simulink model "crazyflie_simulation"  (R2019a)
settings: Solver=FixedStepAuto  StartTime=0.0  StopTime=100  FixedStep=Ts  RelTol=1e-3
undefined symbols (not defined in the file): b, D_0, D_1, D_2, DiscIntNeverNeededParam, g, I_CF_1, I_CF_1_inv, I_rzz, k_f, k_m, kx, ky, kz, l, m_CF, N_0, N_1, N_2, omegaR_init, T, T_init, Ts
libraries: sharedutil x2, simulink x1
settings Model: Creator=evgheniivolodscoi  LastModifiedBy=evgheniivolodscoi

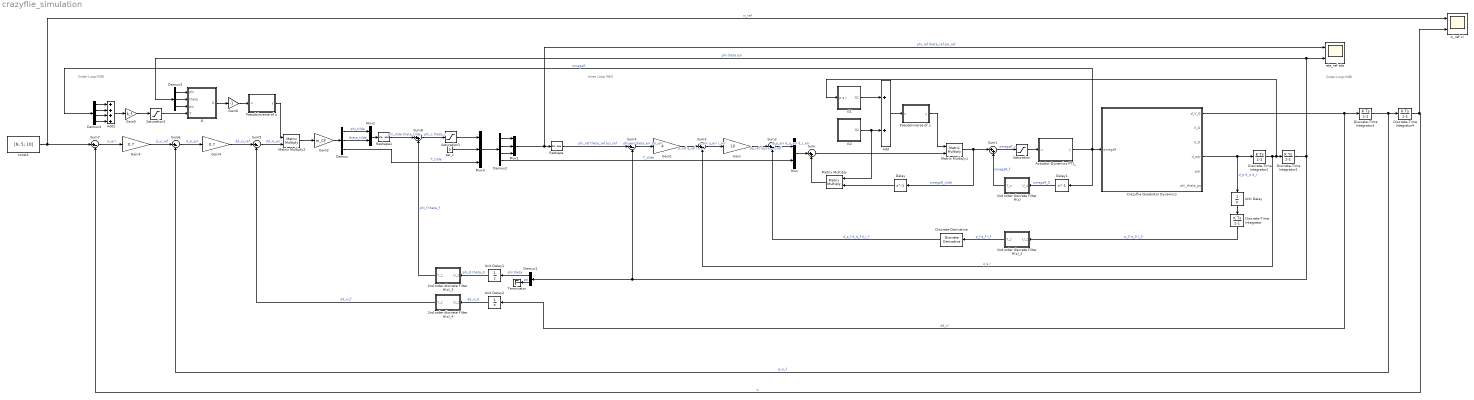
== system crazyflie_simulation ==
  note: Outer Loop INDI
  note: Outer Loop INDI
  note: Inner Loop INDI
  2nd order discrete Filter H(z) : Subsystem
  2nd order discrete Filter H(z)_2 : Subsystem
  2nd order discrete Filter H(z)_3 : Subsystem
  2nd order discrete Filter H(z)_4 : Subsystem
  "Actuator Dynamics PT1_ " : Subsystem
  Add : Sum
  Add1 : Sum  Inputs=++++
  Crazyflie Quadrotor Dynamics : Subsystem
  Delay : Delay  DelayLength=1  InitialCondition=0
  Delay1 : Delay  DelayLength=1  InitialCondition=0
  Demux : Demux  Outputs=3
  Demux1 : Demux  Outputs=2
  Demux2 : Demux
  Demux3 : Demux  Outputs=3
  Demux4 : Demux
  Discrete Derivative : simulink/Discrete/Discrete Derivative  gainval=1.0  ICPrevScaledInput=0.0  OutMin=[]  OutMax=[]  OutDataType=fixdt(1, 16)  OutScaling=2^-10  DoSatur=off
  Discrete-Time Integrator{,1..4} (5 alike) : DiscreteIntegrator  SampleTime=-1  ICPrevOutput=DiscIntNeverNeededParam  ICPrevScaledInput=DiscIntNeverNeededParam
  G : Subsystem
  G1 : Subsystem
  G2 : Subsystem
  Gain : Gain  Gain=10
  Gain1 : Gain  Gain=4
  Gain2 : Gain  Gain=m_CF
  Gain3 : Gain  Gain=0.7
  Gain4 : Gain  Gain=0.7
  Gain5 : Gain  Gain=k_f
  Gain6 : Gain  Gain=-1
  Matrix Multiply : Product  Multiplication=Matrix(*)
  Matrix Multiply1 : Product  Multiplication=Matrix(*)
  Matrix Multiply2 : Product  Multiplication=Matrix(*)
  Mux : Mux  Inputs=2
  Mux1 : Mux  Inputs=3
  Mux2 : Mux  Inputs=2
  Mux3 : Mux  Inputs=3
  Pseudoinverse of u : MATLAB Function  TreatAsAtomicUnit=on
  "Pseudoinverse of u " : MATLAB Function  TreatAsAtomicUnit=on
  Reshape : Reshape  OutputDimensionality=Column vector (2-D)
  Reshape1 : Reshape  OutputDimensionality=Column vector (2-D)
  Saturation : Saturate  UpperLimit=1000  LowerLimit=0
  Saturation1 : Saturate  UpperLimit=60/180*pi  LowerLimit=-60/180*pi
  Saturation2 : Saturate  UpperLimit=inf  LowerLimit=T_init
  Sum : Sum  Inputs=|++
  Sum1 : Sum  Inputs=|++
  Sum{2..7} (6 alike) : Sum  Inputs=|+-
  Sum8 : Sum  Inputs=|++
  Terminator : Terminator
  Unit Delay : UnitDelay  SampleTime=-1  HasFrameUpgradeWarning=on
  Unit Delay1 : UnitDelay  SampleTime=-1  HasFrameUpgradeWarning=on
  Unit Delay2 : UnitDelay  SampleTime=-1  HasFrameUpgradeWarning=on
  const1 : Constant  Value=[6; 5; 10]
  eta_ref eta : Scope  NumInputPorts=2
  psi_c : Constant  Value=0
  xi_ref xi : Scope  NumInputPorts=2
  wires:
  G1/1(G1) -> Add/1
  G2/1(G2) -> Matrix Multiply/1, Add/2
  Matrix Multiply1/1 -> Sum1/1, Delay/1  "omegaR_tilde"
  Delay/1 -> Matrix Multiply/2
  Matrix Multiply/1 -> Sum/2
  Sum/1 -> Matrix Multiply1/2
  Mux/1 -> Sum/1
  Sum1/1 -> Saturation/1  "omegaR_c"
  2nd order discrete Filter H(z)/1(Y_z) -> Sum1/2  "omegaR_f"
  Delay1/1 -> 2nd order discrete Filter H(z)/1(U_z)  "omegaR_0"
  "Actuator Dynamics PT1_ "/1(y) -> Demux4/1, Delay1/1, Crazyflie Quadrotor Dynamics/1(omegaR)  "omegaR"
  Add/1 -> Pseudoinverse of u/1(u)
  Sum2/1 -> Mux/1  "d_p_err d_q_err d_r_err"
  Discrete Derivative/1 -> Sum2/2  "d_p_f d_q_f d_r_f"
  Gain/1 -> Sum2/1  "dp_ref dq_ref dr_ref"
  Sum3/1 -> Gain/1  "p_err q_err r_err"
  Gain1/1 -> Sum3/1  "p_ref q_ref r_ref"
  Discrete-Time Integrator1/1 -> Sum3/2, G1/1(p q r), Discrete-Time Integrator2/1  "p q r"
  Sum4/1 -> Gain1/1  "phi_err theta_err psi_err"
  Discrete-Time Integrator/1 -> 2nd order discrete Filter H(z)_2/1(U_z)  "p_0 q_0 r_0"
  2nd order discrete Filter H(z)_2/1(Y_z) -> Discrete Derivative/1  "p_f q_f r_f"
  Crazyflie Quadrotor Dynamics/4(d_pqr) -> Discrete-Time Integrator1/1, Unit Delay/1  "d_p d_q d_r"
  Unit Delay/1 -> Discrete-Time Integrator/1
  Gain2/1 -> Demux/1
  Sum5/1 -> Matrix Multiply2/2  "dd_xi_err"
  Gain4/1 -> Sum5/1  "dd_xi_ref"
  Gain3/1 -> Sum6/1  "d_xi_ref"
  Sum7/1 -> Gain3/1  "xi_err"
  Discrete-Time Integrator4/1 -> xi_ref xi/2, Sum7/2  "xi"
  const1/1 -> Sum7/1, xi_ref xi/1  "xi_ref"
  Matrix Multiply2/1 -> Gain2/1
  Reshape1/1 -> Sum8/1  "phi_tilde theta_tilde"
  2nd order discrete Filter H(z)_3/1(Y_z) -> Sum8/2  "phi_f theta_f"
  Sum8/1 -> Saturation1/1  "phi_c theta_c"
  Unit Delay1/1 -> 2nd order discrete Filter H(z)_3/1(U_z)  "phi_0 theta_0"
  Demux1/1 -> Unit Delay1/1  "phi theta"
  Demux1/2 -> Terminator/1  "psi"
  Crazyflie Quadrotor Dynamics/1(d_V_O) -> Unit Delay2/1, Discrete-Time Integrator3/1  "dd_xi"
  Discrete-Time Integrator2/1 -> eta_ref eta/2, Demux3/1, Demux1/1, Sum4/2  "phi theta psi"
  Mux1/1 -> eta_ref eta/1, Reshape/1  "phi_ref theta_ref psi_ref"
  Demux2/2 -> Mux1/2
  Demux2/1 -> Mux1/1
  Demux2/3 -> Mux1/3
  Demux2/4 -> Mux/2  "T_tilde"
  Reshape/1 -> Sum4/1  "phi_ref theta_ref psi_ref"
  Pseudoinverse of u/1(y) -> Matrix Multiply1/1
  Demux/1 -> Mux2/1  "phi_tilde"
  Demux/2 -> Mux2/2  "theta_tilde"
  Demux/3 -> Mux3/3  "T_tilde"
  Mux2/1 -> Reshape1/1
  psi_c/1 -> Mux3/2
  Mux3/1 -> Demux2/1
  "Pseudoinverse of u "/1(y) -> Matrix Multiply2/1
  Demux3/1 -> G/1(phi)
  Demux3/2 -> G/2(theta)
  Demux3/3 -> G/3(psi)
  Demux4/1 -> Add1/1
  Demux4/2 -> Add1/2
  Demux4/3 -> Add1/3
  Demux4/4 -> Add1/4
  Add1/1 -> Gain5/1
  Gain5/1 -> Saturation2/1
  2nd order discrete Filter H(z)_4/1(Y_z) -> Sum5/2  "dd_xi_f"
  Unit Delay2/1 -> 2nd order discrete Filter H(z)_4/1(U_z)  "dd_xi_0"
  Discrete-Time Integrator3/1 -> Sum6/2, Discrete-Time Integrator4/1  "d_xi_f"
  Sum6/1 -> Gain4/1  "d_xi_err"
  G/1(G) -> Gain6/1
  Saturation/1 -> "Actuator Dynamics PT1_ "/1(u)
  Saturation1/1 -> Mux3/1
  Saturation2/1 -> G/4(T)
  Gain6/1 -> "Pseudoinverse of u "/1(u)

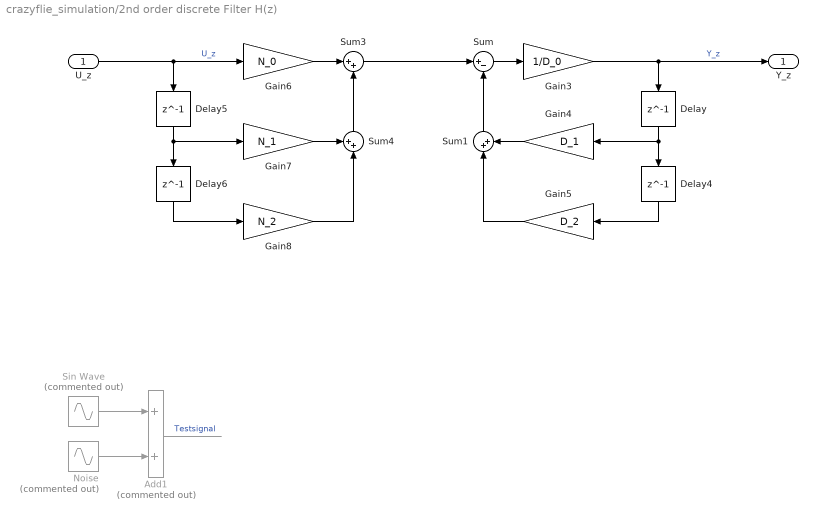
== system crazyflie_simulation/2nd order discrete Filter H(z) ==
  U_z : Inport
  Add1 : Sum  Commented=on
  Delay{,4..6} (4 alike) : Delay  DelayLength=1  InitialCondition=0
  Gain3 : Gain  Gain=1/D_0
  Gain4 : Gain  Gain=D_1
  Gain5 : Gain  Gain=D_2
  Gain6 : Gain  Gain=N_0
  Gain7 : Gain  Gain=N_1
  Gain8 : Gain  Gain=N_2
  Noise : Sin  Commented=on  Amplitude=0.15  Frequency=10*2*pi  SampleTime=0
  Sin Wave : Sin  Commented=on  Frequency=100/2/pi*2*pi  SampleTime=0
  Sum : Sum  Inputs=|+-
  Sum1 : Sum  Inputs=|++
  Sum3 : Sum  Inputs=|++
  Sum4 : Sum  Inputs=++|
  Y_z : Outport
  wires:
  Add1/1 -> ?  "Testsignal"
  Sin Wave/1 -> Add1/1
  Noise/1 -> Add1/2
  Delay6/1 -> Gain8/1
  Gain8/1 -> Sum4/2
  Sum4/1 -> Sum3/2
  Gain7/1 -> Sum4/1
  Delay5/1 -> Gain7/1, Delay6/1
  U_z/1 -> Gain6/1, Delay5/1  "U_z"
  Gain6/1 -> Sum3/1
  Sum3/1 -> Sum/1
  Gain5/1 -> Sum1/1
  Gain4/1 -> Sum1/2
  Gain3/1 -> Delay/1, Y_z/1  "Y_z"
  Sum1/1 -> Sum/2
  Delay4/1 -> Gain5/1
  Delay/1 -> Gain4/1, Delay4/1
  Sum/1 -> Gain3/1

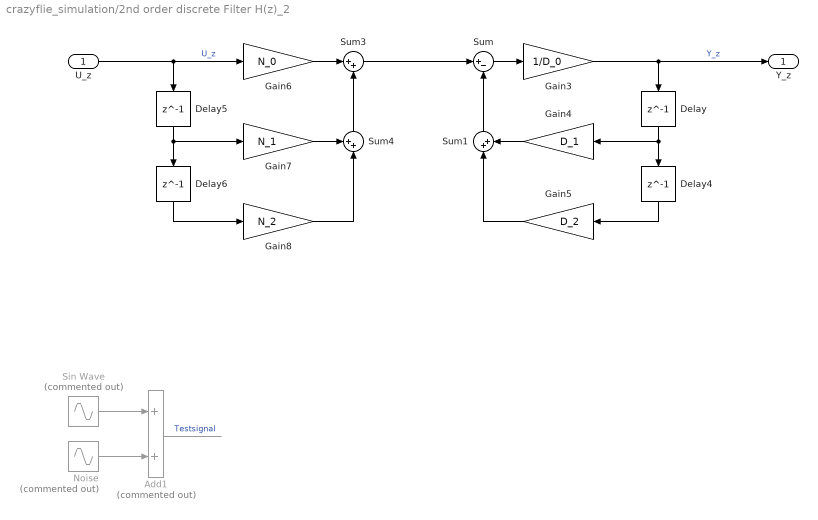
== system crazyflie_simulation/2nd order discrete Filter H(z)_2 ==
  U_z : Inport
  Add1 : Sum  Commented=on
  Delay{,4..6} (4 alike) : Delay  DelayLength=1  InitialCondition=0
  Gain3 : Gain  Gain=1/D_0
  Gain4 : Gain  Gain=D_1
  Gain5 : Gain  Gain=D_2
  Gain6 : Gain  Gain=N_0
  Gain7 : Gain  Gain=N_1
  Gain8 : Gain  Gain=N_2
  Noise : Sin  Commented=on  Amplitude=0.15  Frequency=10*2*pi  SampleTime=0
  Sin Wave : Sin  Commented=on  Frequency=100/2/pi*2*pi  SampleTime=0
  Sum : Sum  Inputs=|+-
  Sum1 : Sum  Inputs=|++
  Sum3 : Sum  Inputs=|++
  Sum4 : Sum  Inputs=++|
  Y_z : Outport
  wires:
  Sum/1 -> Gain3/1
  Delay/1 -> Delay4/1, Gain4/1
  Delay4/1 -> Gain5/1
  Sum1/1 -> Sum/2
  Gain3/1 -> Y_z/1, Delay/1  "Y_z"
  Gain4/1 -> Sum1/2
  Gain5/1 -> Sum1/1
  Sum3/1 -> Sum/1
  Gain6/1 -> Sum3/1
  U_z/1 -> Delay5/1, Gain6/1  "U_z"
  Delay5/1 -> Delay6/1, Gain7/1
  Gain7/1 -> Sum4/1
  Sum4/1 -> Sum3/2
  Gain8/1 -> Sum4/2
  Delay6/1 -> Gain8/1
  Noise/1 -> Add1/2
  Sin Wave/1 -> Add1/1
  Add1/1 -> ?  "Testsignal"

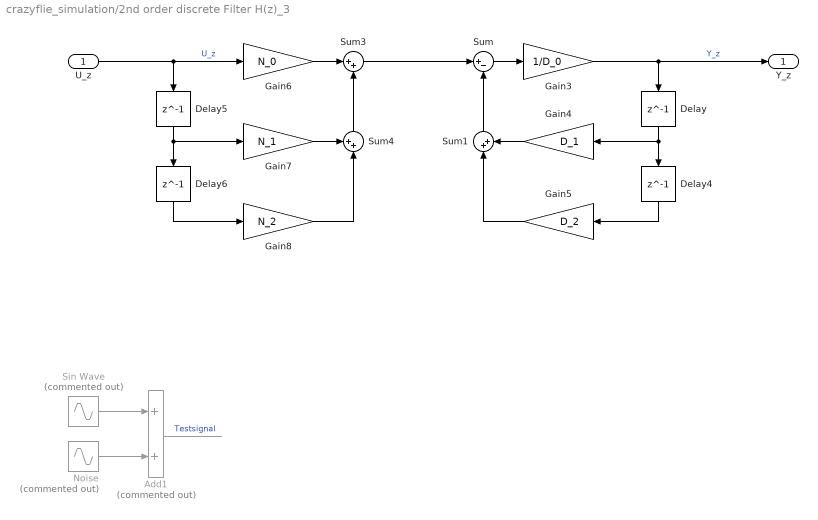
== system crazyflie_simulation/2nd order discrete Filter H(z)_3 ==
  U_z : Inport
  Add1 : Sum  Commented=on
  Delay{,4..6} (4 alike) : Delay  DelayLength=1  InitialCondition=0
  Gain3 : Gain  Gain=1/D_0
  Gain4 : Gain  Gain=D_1
  Gain5 : Gain  Gain=D_2
  Gain6 : Gain  Gain=N_0
  Gain7 : Gain  Gain=N_1
  Gain8 : Gain  Gain=N_2
  Noise : Sin  Commented=on  Amplitude=0.15  Frequency=10*2*pi  SampleTime=0
  Sin Wave : Sin  Commented=on  Frequency=100/2/pi*2*pi  SampleTime=0
  Sum : Sum  Inputs=|+-
  Sum1 : Sum  Inputs=|++
  Sum3 : Sum  Inputs=|++
  Sum4 : Sum  Inputs=++|
  Y_z : Outport
  wires:
  Add1/1 -> ?  "Testsignal"
  Sin Wave/1 -> Add1/1
  Noise/1 -> Add1/2
  Delay6/1 -> Gain8/1
  Gain8/1 -> Sum4/2
  Sum4/1 -> Sum3/2
  Gain7/1 -> Sum4/1
  Delay5/1 -> Gain7/1, Delay6/1
  U_z/1 -> Gain6/1, Delay5/1  "U_z"
  Gain6/1 -> Sum3/1
  Sum3/1 -> Sum/1
  Gain5/1 -> Sum1/1
  Gain4/1 -> Sum1/2
  Gain3/1 -> Delay/1, Y_z/1  "Y_z"
  Sum1/1 -> Sum/2
  Delay4/1 -> Gain5/1
  Delay/1 -> Gain4/1, Delay4/1
  Sum/1 -> Gain3/1

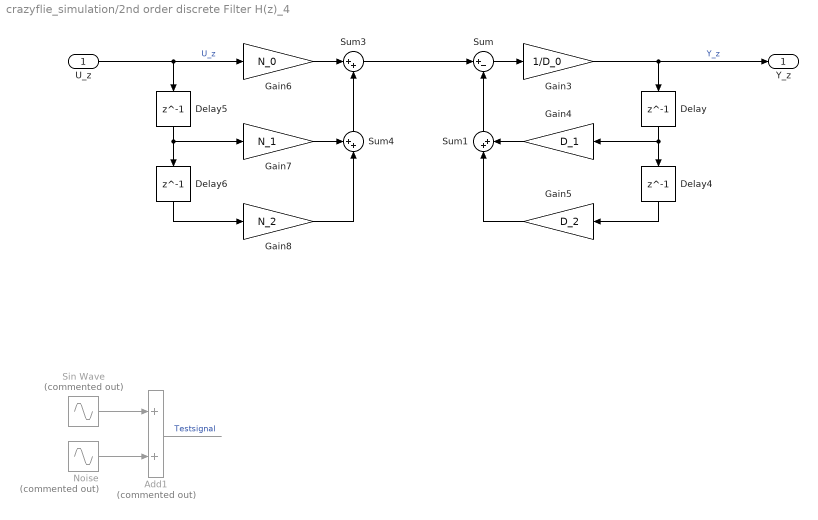
== system crazyflie_simulation/2nd order discrete Filter H(z)_4 ==
  U_z : Inport
  Add1 : Sum  Commented=on
  Delay{,4..6} (4 alike) : Delay  DelayLength=1  InitialCondition=0
  Gain3 : Gain  Gain=1/D_0
  Gain4 : Gain  Gain=D_1
  Gain5 : Gain  Gain=D_2
  Gain6 : Gain  Gain=N_0
  Gain7 : Gain  Gain=N_1
  Gain8 : Gain  Gain=N_2
  Noise : Sin  Commented=on  Amplitude=0.15  Frequency=10*2*pi  SampleTime=0
  Sin Wave : Sin  Commented=on  Frequency=100/2/pi*2*pi  SampleTime=0
  Sum : Sum  Inputs=|+-
  Sum1 : Sum  Inputs=|++
  Sum3 : Sum  Inputs=|++
  Sum4 : Sum  Inputs=++|
  Y_z : Outport
  wires:
  Sum/1 -> Gain3/1
  Delay/1 -> Delay4/1, Gain4/1
  Delay4/1 -> Gain5/1
  Sum1/1 -> Sum/2
  Gain3/1 -> Y_z/1, Delay/1  "Y_z"
  Gain4/1 -> Sum1/2
  Gain5/1 -> Sum1/1
  Sum3/1 -> Sum/1
  Gain6/1 -> Sum3/1
  U_z/1 -> Delay5/1, Gain6/1  "U_z"
  Delay5/1 -> Delay6/1, Gain7/1
  Gain7/1 -> Sum4/1
  Sum4/1 -> Sum3/2
  Gain8/1 -> Sum4/2
  Delay6/1 -> Gain8/1
  Noise/1 -> Add1/2
  Sin Wave/1 -> Add1/1
  Add1/1 -> ?  "Testsignal"

== system crazyflie_simulation/Actuator Dynamics PT1_  ==
  u : Inport
  Gain : Gain  Gain=1/T
  Integrator : Integrator  InitialCondition=omegaR_init
  Sum : Sum  Inputs=|+-
  y : Outport
  wires:
  Sum/1 -> Gain/1
  Gain/1 -> Integrator/1  "d_y"
  u/1 -> Sum/1
  Integrator/1 -> y/1, Sum/2  "y"

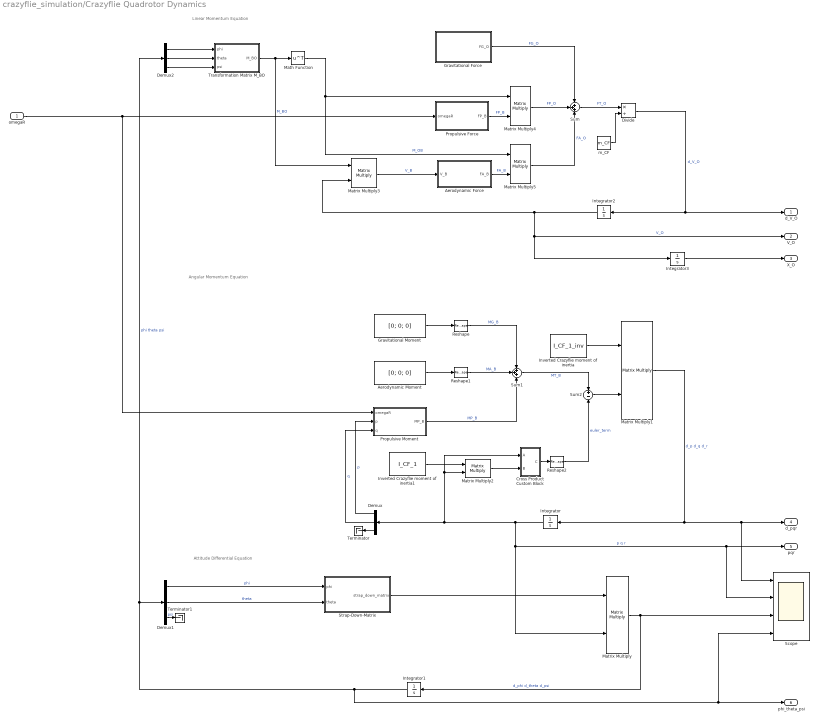
== system crazyflie_simulation/Crazyflie Quadrotor Dynamics ==
  note: Attitude Differential Equation
  note: Angular Momentum Equation
  note: Linear Momentum Equation
  omegaR : Inport
  Aerodynamic Force : Subsystem
  Aerodynamic Moment : Constant  Value=[0; 0; 0]
  Cross Product Custom Block : Subsystem
  Demux : Demux  Outputs=3
  Demux1 : Demux  Outputs=3
  Demux2 : Demux  Outputs=3
  Divide : Product  Inputs=*/
  "Gravitational Force " : Subsystem
  Gravitational Moment : Constant  Value=[0; 0; 0]
  Integrator{,1..3} (4 alike) : Integrator  InitialCondition=[0; 0; 0]
  Inverted Crazyflie moment of inertia : Constant  Value=I_CF_1_inv
  Inverted Crazyflie moment of inertia1 : Constant  Value=I_CF_1
  Math Function : Math  Operator=transpose  SaturateOnIntegerOverflow=on
  Matrix Multiply{,1..5} (6 alike) : Product  Multiplication=Matrix(*)
  Propulsive Force : Subsystem
  Propulsive Moment : Subsystem
  Reshape : Reshape  OutputDimensionality=Column vector (2-D)
  Reshape1 : Reshape  OutputDimensionality=Column vector (2-D)
  Reshape2 : Reshape  OutputDimensionality=Column vector (2-D)
  Scope : Scope  NumInputPorts=4
  Strap-Down-Matrix : Subsystem
  Sum : Sum  Inputs=+++
  Sum1 : Sum  Inputs=+++
  Sum2 : Sum  Inputs=+-
  Terminator : Terminator
  Terminator1 : Terminator
  Transformation Matrix M_BO : Subsystem
  m_CF : Constant  Value=m_CF
  d_V_O : Outport
  V_O : Outport  Port=2
  X_O : Outport  Port=3
  d_pqr : Outport  Port=4
  pqr : Outport  Port=5
  phi_theta_psi : Outport  Port=6
  wires:
  Inverted Crazyflie moment of inertia1/1 -> Matrix Multiply2/1
  Sum2/1 -> Matrix Multiply1/2
  Integrator3/1 -> X_O/1
  Integrator2/1 -> Matrix Multiply3/2, V_O/1, Integrator3/1  "V_O"
  Divide/1 -> Integrator2/1, d_V_O/1  "d_V_O"
  omegaR/1 -> Propulsive Force/1(omegaR), Propulsive Moment/1(omegaR)
  Reshape2/1 -> Sum2/2  "euler_term"
  Reshape1/1 -> Sum1/2  "MA_B"
  Reshape/1 -> Sum1/1  "MG_B"
  Demux/2 -> Propulsive Moment/3(q)  "q"
  Sum1/1 -> Sum2/1  "MT_B"
  Demux1/1 -> Strap-Down-Matrix/1(phi)  "phi"
  Demux2/3 -> Transformation Matrix M_BO/3(psi)
  Strap-Down-Matrix/1(strap_down_matrix) -> Matrix Multiply/1
  Matrix Multiply5/1 -> Sum/3  "FA_O"
  Math Function/1 -> Matrix Multiply5/1, Matrix Multiply4/1  "M_OB"
  Demux2/1 -> Transformation Matrix M_BO/1(phi)
  Matrix Multiply3/1 -> Aerodynamic Force/1(V_B)  "V_B"
  Matrix Multiply/1 -> Scope/3, Integrator1/1  "d_phi d_theta d_psi"
  Cross Product Custom Block/1(C) -> Reshape2/1
  Matrix Multiply2/1 -> Cross Product Custom Block/2(B)
  Aerodynamic Force/1(FA_B) -> Matrix Multiply5/2  "FA_B"
  Transformation Matrix M_BO/1(M_BO) -> Math Function/1, Matrix Multiply3/1  "M_BO"
  Gravitational Moment/1 -> Reshape/1
  m_CF/1 -> Divide/2
  Demux2/2 -> Transformation Matrix M_BO/2(theta)
  Sum/1 -> Divide/1  "FT_O"
  Propulsive Moment/1(MP_B) -> Sum1/3  "MP_B"
  Matrix Multiply4/1 -> Sum/2  "FP_O"
  "Gravitational Force "/1(FG_O) -> Sum/1  "FG_O"
  Propulsive Force/1(FP_B) -> Matrix Multiply4/2  "FP_B"
  Integrator/1 -> pqr/1, Scope/2, Matrix Multiply/2, Matrix Multiply2/2, Cross Product Custom Block/1(A), Demux/1  "p q r"
  Demux/1 -> Propulsive Moment/2(p)  "p"
  Integrator1/1 -> phi_theta_psi/1, Scope/4, Demux1/1, Demux2/1  "phi theta psi"
  Inverted Crazyflie moment of inertia/1 -> Matrix Multiply1/1
  Demux1/2 -> Strap-Down-Matrix/2(theta)  "theta"
  Matrix Multiply1/1 -> d_pqr/1, Scope/1, Integrator/1  "d_p d_q d_r"
  Aerodynamic Moment/1 -> Reshape1/1
  Demux/3 -> Terminator/1
  Demux1/3 -> Terminator1/1  "psi"

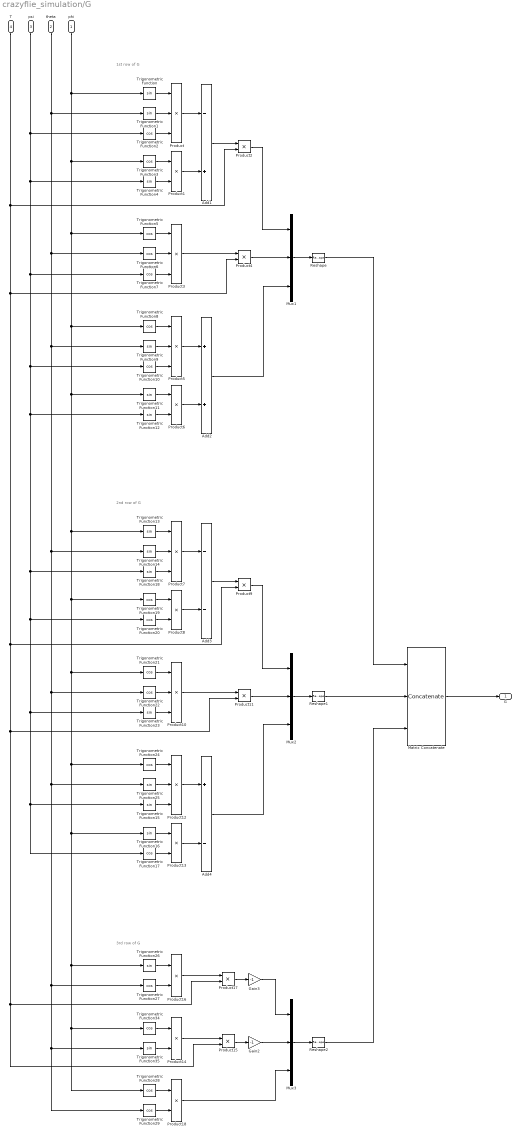
== system crazyflie_simulation/G ==
  note: 1st row of G
  note: 2nd row of G
  note: 3rd row of G
  phi : Inport
  theta : Inport  Port=2
  psi : Inport  Port=3
  T : Inport  Port=4
  Add1 : Sum  Inputs=-+
  Add2 : Sum
  Add3 : Sum  Inputs=--
  Add4 : Sum  Inputs=+-
  Gain2 : Gain  Gain=-1
  Gain3 : Gain  Gain=-1
  Matrix Concatenate : Concatenate  NumInputs=3  Mode=Multidimensional array
  Mux1 : Mux  Inputs=3
  Mux2 : Mux  Inputs=3
  Mux3 : Mux  Inputs=3
  Product{,3,5,7,10,12} (6 alike) : Product  Inputs=3
  Product{1..2,4,6,8..9,11,13..18} (13 alike) : Product
  Reshape : Reshape  OutputDimensionality=Row vector (2-D)
  Reshape1 : Reshape  OutputDimensionality=Row vector (2-D)
  Reshape2 : Reshape  OutputDimensionality=Row vector (2-D)
  Trigonometric Function{,1,4,9,11..16,18,23,25..26,35} (15 alike) : Trigonometry
  Trigonometric Function{2..3,5..8,10,17,19..22,24,27..29,34} (17 alike) : Trigonometry  Operator=cos
  G : Outport
  wires:
  T/1 -> Product2/2, Product4/2, Product9/2, Product11/2, Product17/2, Product15/2
  Mux1/1 -> Reshape/1
  theta/1 -> Trigonometric Function1/1, Trigonometric Function6/1, Trigonometric Function9/1, Trigonometric Function14/1, Trigonometric Function22/1, Trigonometric Function25/1, Trigonometric Function27/1, Trigonometric Function35/1, Trigonometric Function29/1
  Trigonometric Function34/1 -> Product14/1
  Reshape/1 -> Matrix Concatenate/1
  psi/1 -> Trigonometric Function2/1, Trigonometric Function4/1, Trigonometric Function7/1, Trigonometric Function10/1, Trigonometric Function12/1, Trigonometric Function18/1, Trigonometric Function20/1, Trigonometric Function23/1, Trigonometric Function15/1, Trigonometric Function17/1
  Trigonometric Function25/1 -> Product12/2
  Trigonometric Function26/1 -> Product16/1
  Add1/1 -> Product2/1
  phi/1 -> Trigonometric Function3/1, Trigonometric Function8/1, Trigonometric Function13/1, Trigonometric Function19/1, Trigonometric Function21/1, Trigonometric Function24/1, Trigonometric Function26/1, Trigonometric Function34/1, Trigonometric Function28/1, Trigonometric Function16/1, Trigonometric Function11/1, Trigonometric Function5/1, Trigonometric Function/1
  Trigonometric Function15/1 -> Product12/3
  Trigonometric Function24/1 -> Product12/1
  Trigonometric Function20/1 -> Product8/2
  Product18/1 -> Mux3/3
  Product4/1 -> Mux1/2
  Mux3/1 -> Reshape2/1
  Product7/1 -> Add3/1
  Trigonometric Function6/1 -> Product3/2
  Matrix Concatenate/1 -> G/1
  Trigonometric Function7/1 -> Product3/3
  Trigonometric Function3/1 -> Product1/1
  Trigonometric Function29/1 -> Product18/2
  Trigonometric Function5/1 -> Product3/1
  Product1/1 -> Add1/2
  Trigonometric Function8/1 -> Product5/1
  Product6/1 -> Add2/2
  Product15/1 -> Gain2/1
  Mux2/1 -> Reshape1/1
  Product17/1 -> Gain3/1
  Gain2/1 -> Mux3/2
  Trigonometric Function17/1 -> Product13/2
  Product12/1 -> Add4/1
  Trigonometric Function19/1 -> Product8/1
  Product3/1 -> Product4/1
  Product9/1 -> Mux2/1
  Product16/1 -> Product17/1
  Add4/1 -> Mux2/3
  Trigonometric Function16/1 -> Product13/1
  Product8/1 -> Add3/2
  Trigonometric Function13/1 -> Product7/1
  Trigonometric Function28/1 -> Product18/1
  Gain3/1 -> Mux3/1
  Add3/1 -> Product9/1
  Trigonometric Function35/1 -> Product14/2
  Trigonometric Function18/1 -> Product7/3
  Product14/1 -> Product15/1
  Trigonometric Function/1 -> Product/1
  Product11/1 -> Mux2/2
  Product13/1 -> Add4/2
  Trigonometric Function21/1 -> Product10/1
  Product10/1 -> Product11/1
  Trigonometric Function22/1 -> Product10/2
  Trigonometric Function23/1 -> Product10/3
  Trigonometric Function14/1 -> Product7/2
  Reshape2/1 -> Matrix Concatenate/3
  Trigonometric Function1/1 -> Product/2
  Product2/1 -> Mux1/1
  Trigonometric Function11/1 -> Product6/1
  Trigonometric Function4/1 -> Product1/2
  Add2/1 -> Mux1/3
  Product5/1 -> Add2/1
  Trigonometric Function2/1 -> Product/3
  Trigonometric Function27/1 -> Product16/2
  Trigonometric Function12/1 -> Product6/2
  Trigonometric Function9/1 -> Product5/2
  Trigonometric Function10/1 -> Product5/3
  Product/1 -> Add1/1
  Reshape1/1 -> Matrix Concatenate/2

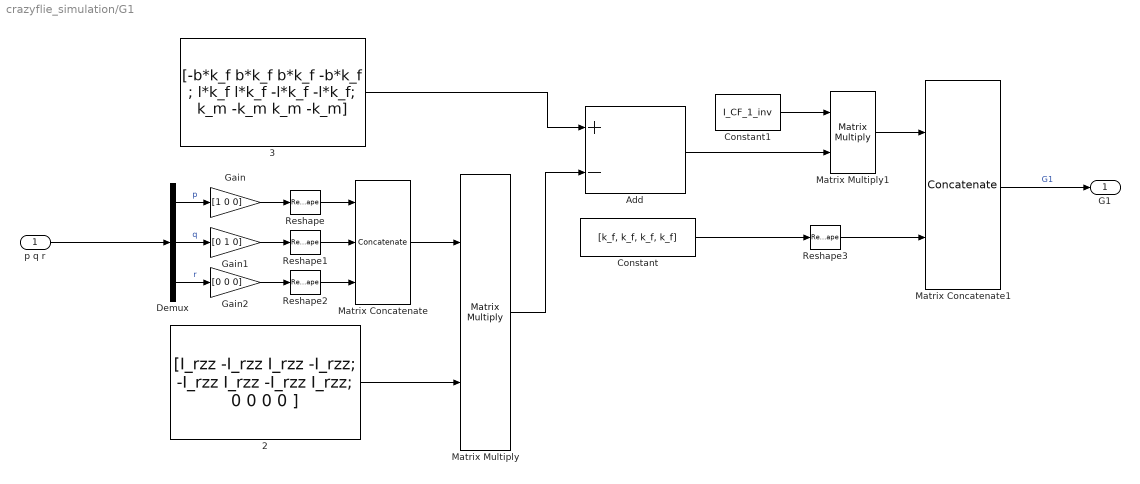
== system crazyflie_simulation/G1 ==
  p q r : Inport
  "  2" : Constant  Value=[I_rzz -I_rzz I_rzz -I_rzz; -I_rzz I_rzz -I_rzz I_rzz; 0 0 0 0 ]
  "  3" : Constant  Value=|
      | [-b*k_f  b*k_f  b*k_f  -b*k_f
      | ;  l*k_f  l*k_f -l*k_f  -l*k_f; k_m   -k_m    k_m    -k_m]
  Add : Sum  Inputs=+-
  Constant : Constant  Value=[k_f, k_f, k_f, k_f]
  Constant1 : Constant  Value=I_CF_1_inv
  Demux : Demux  Outputs=3
  Gain : Gain  Gain=[1 0 0]
  Gain1 : Gain  Gain=[0 1 0]
  Gain2 : Gain  Gain=[0 0 0]
  Matrix Concatenate : Concatenate  NumInputs=3  Mode=Multidimensional array
  Matrix Concatenate1 : Concatenate  Mode=Multidimensional array
  Matrix Multiply : Product  Multiplication=Matrix(*)
  Matrix Multiply1 : Product  Multiplication=Matrix(*)
  Reshape{,1..3} (4 alike) : Reshape  OutputDimensionality=Row vector (2-D)
  G1 : Outport
  wires:
  Demux/1 -> Gain/1  "p"
  Gain/1 -> Reshape/1
  Matrix Concatenate/1 -> Matrix Multiply/1
  Demux/2 -> Gain1/1  "q"
  Reshape1/1 -> Matrix Concatenate/2
  Constant/1 -> Reshape3/1
  Reshape2/1 -> Matrix Concatenate/3
  Add/1 -> Matrix Multiply1/2
  Gain2/1 -> Reshape2/1
  "  2"/1 -> Matrix Multiply/2
  Reshape3/1 -> Matrix Concatenate1/2
  Matrix Multiply/1 -> Add/2
  "  3"/1 -> Add/1
  Gain1/1 -> Reshape1/1
  Demux/3 -> Gain2/1  "r"
  Reshape/1 -> Matrix Concatenate/1
  Matrix Concatenate1/1 -> G1/1  "G1"
  p q r/1 -> Demux/1
  Matrix Multiply1/1 -> Matrix Concatenate1/1
  Constant1/1 -> Matrix Multiply1/1

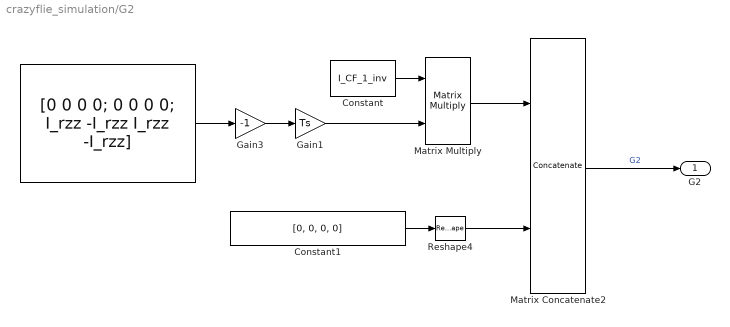
== system crazyflie_simulation/G2 ==
  "  " : Constant  Value=[0 0 0 0; 0 0 0 0; I_rzz -I_rzz I_rzz -I_rzz]
  Constant : Constant  Value=I_CF_1_inv
  Constant1 : Constant  Value=[0, 0, 0, 0]
  Gain1 : Gain  Gain=Ts
  Gain3 : Gain  Gain=-1
  Matrix Concatenate2 : Concatenate  Mode=Multidimensional array
  Matrix Multiply : Product  Multiplication=Matrix(*)
  Reshape4 : Reshape  OutputDimensionality=Row vector (2-D)
  G2 : Outport
  wires:
  Gain3/1 -> Gain1/1
  "  "/1 -> Gain3/1
  Reshape4/1 -> Matrix Concatenate2/2
  Constant1/1 -> Reshape4/1
  Matrix Concatenate2/1 -> G2/1  "G2"
  Gain1/1 -> Matrix Multiply/2
  Constant/1 -> Matrix Multiply/1
  Matrix Multiply/1 -> Matrix Concatenate2/1

== system crazyflie_simulation/Crazyflie Quadrotor Dynamics/Aerodynamic Force ==
  V_B : Inport
  Demux : Demux  Outputs=3
  Gain : Gain  Gain=-kx
  Gain1 : Gain  Gain=-ky
  Gain2 : Gain  Gain=-kz
  Mux1 : Mux  Inputs=3
  Reshape : Reshape  OutputDimensionality=Column vector (2-D)
  FA_B : Outport
  wires:
  Reshape/1 -> FA_B/1  "FA_B"
  Demux/1 -> Gain/1  "v_B"
  Demux/3 -> Gain2/1  "w_B"
  V_B/1 -> Demux/1
  Demux/2 -> Gain1/1  "u_B"
  Gain/1 -> Mux1/1
  Gain1/1 -> Mux1/2
  Mux1/1 -> Reshape/1
  Gain2/1 -> Mux1/3

== system crazyflie_simulation/Crazyflie Quadrotor Dynamics/Cross Product Custom Block ==
  A : Inport
  B : Inport  Port=2
  A1 : InportShadow
  B1 : InportShadow  Port=2
  Subsystem : sharedutil/3x3 Cross Product/Subsystem  SystemSampleTime=-1
      settings: SourceProductName=Aerospace Blockset  SourceProductBaseCode=AE
  Subsystem1 : sharedutil/3x3 Cross Product/Subsystem1  SystemSampleTime=-1
      settings: SourceProductName=Aerospace Blockset  SourceProductBaseCode=AE
  Sum3 : Sum  Inputs=+|-  SaturateOnIntegerOverflow=on  InputSameDT=on  OutDataTypeStr=Inherit: Same as first input
  C : Outport
  wires:
  Subsystem/1 -> Sum3/1
  B1/1 -> Subsystem1/2
  Sum3/1 -> C/1
  B/1 -> Subsystem/2
  Subsystem1/1 -> Sum3/2
  A/1 -> Subsystem/1
  A1/1 -> Subsystem1/1

== system crazyflie_simulation/Crazyflie Quadrotor Dynamics/Gravitational Force  ==
  Product : Product
  Reshape : Reshape  OutputDimensionality=Column vector (2-D)
  g_acc : Constant  Value=[0; 0; g]
  m_CF : Constant  Value=m_CF
  FG_O : Outport
  wires:
  Reshape/1 -> FG_O/1  "FG_O"
  Product/1 -> Reshape/1
  g_acc/1 -> Product/1
  m_CF/1 -> Product/2

== system crazyflie_simulation/Crazyflie Quadrotor Dynamics/Propulsive Force ==
  omegaR : Inport
  Constant : Constant  Value=0
  Demux1 : Demux
  Gain4 : Gain  Gain=-k_f
  Matrix Sum2 : Sum  Inputs=++++
  Mux : Mux  Inputs=3
  Reshape : Reshape  OutputDimensionality=Column vector (2-D)
  FP_B : Outport
  wires:
  Constant/1 -> Mux/1, Mux/2
  Reshape/1 -> FP_B/1  "FP_B"
  Demux1/3 -> Matrix Sum2/3  "omegaR_3"
  Demux1/1 -> Matrix Sum2/1  "omegaR_1"
  Demux1/4 -> Matrix Sum2/4  "omegaR_4"
  Mux/1 -> Reshape/1
  Matrix Sum2/1 -> Gain4/1
  omegaR/1 -> Demux1/1
  Demux1/2 -> Matrix Sum2/2  "omegaR_2"
  Gain4/1 -> Mux/3

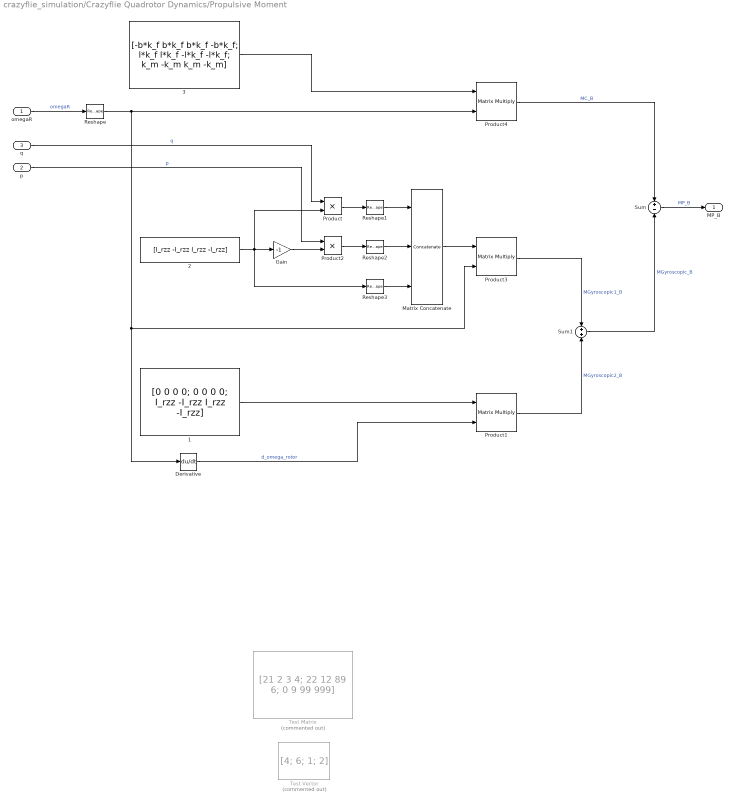
== system crazyflie_simulation/Crazyflie Quadrotor Dynamics/Propulsive Moment ==
  omegaR : Inport
  p : Inport  Port=2
  q : Inport  Port=3
  "  1" : Constant  Value=[0 0 0 0; 0 0 0 0; I_rzz -I_rzz I_rzz -I_rzz]
  "  2" : Constant  Value=[I_rzz -I_rzz I_rzz -I_rzz]
  "  3" : Constant  Value=[-b*k_f b*k_f b*k_f -b*k_f; l*k_f l*k_f -l*k_f -l*k_f; k_m -k_m k_m -k_m]
  "  Test Matrix" : Constant  Commented=on  Value=[21 2 3 4; 22 12 89 6; 0 9 99 999]
  Derivative : Derivative
  Gain : Gain  Gain=-1
  Matrix Concatenate : Concatenate  NumInputs=3  Mode=Multidimensional array
  Product : Product
  Product1 : Product  Multiplication=Matrix(*)
  Product2 : Product
  Product3 : Product  Multiplication=Matrix(*)
  Product4 : Product  Multiplication=Matrix(*)
  Reshape : Reshape  OutputDimensionality=Column vector (2-D)
  Reshape1 : Reshape  OutputDimensionality=Row vector (2-D)
  Reshape2 : Reshape  OutputDimensionality=Row vector (2-D)
  Reshape3 : Reshape  OutputDimensionality=Row vector (2-D)
  Sum : Sum  Inputs=+-
  Sum1 : Sum
  Test Vector : Constant  Commented=on  Value=[4; 6; 1; 2]
  MP_B : Outport
  wires:
  Matrix Concatenate/1 -> Product3/1
  "  3"/1 -> Product4/1
  Reshape/1 -> Product3/2, Derivative/1, Product4/2
  q/1 -> Product/1  "q"
  Gain/1 -> Product2/2
  Product1/1 -> Sum1/2  "MGyroscopic2_B"
  Derivative/1 -> Product1/2  "d_omega_rotor"
  "  1"/1 -> Product1/1
  Product3/1 -> Sum1/1  "MGyroscopic1_B"
  p/1 -> Product2/1  "p"
  "  2"/1 -> Product/2, Gain/1, Reshape3/1
  Product2/1 -> Reshape2/1
  Product/1 -> Reshape1/1
  Sum1/1 -> Sum/2  "MGyroscopic_B"
  Sum/1 -> MP_B/1  "MP_B"
  Product4/1 -> Sum/1  "MC_B"
  omegaR/1 -> Reshape/1  "omegaR"
  Reshape1/1 -> Matrix Concatenate/1
  Reshape2/1 -> Matrix Concatenate/2
  Reshape3/1 -> Matrix Concatenate/3

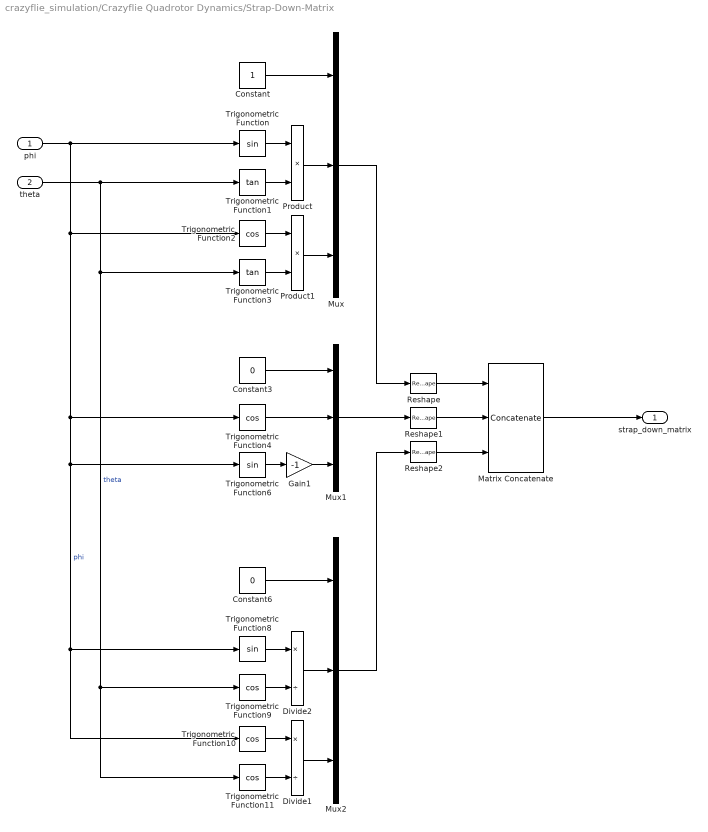
== system crazyflie_simulation/Crazyflie Quadrotor Dynamics/Strap-Down-Matrix ==
  phi : Inport
  theta : Inport  Port=2
  Constant : Constant
  Constant3 : Constant  Value=0
  Constant6 : Constant  Value=0
  Divide1 : Product  Inputs=*/
  Divide2 : Product  Inputs=*/
  Gain1 : Gain  Gain=-1
  Matrix Concatenate : Concatenate  NumInputs=3  Mode=Multidimensional array
  Mux : Mux  Inputs=3
  Mux1 : Mux  Inputs=3
  Mux2 : Mux  Inputs=3
  Product : Product
  Product1 : Product
  Reshape : Reshape  OutputDimensionality=Row vector (2-D)
  Reshape1 : Reshape  OutputDimensionality=Row vector (2-D)
  Reshape2 : Reshape  OutputDimensionality=Row vector (2-D)
  Trigonometric Function : Trigonometry
  Trigonometric Function1 : Trigonometry  Operator=tan
  Trigonometric Function{2,4,9..11} (5 alike) : Trigonometry  Operator=cos
  Trigonometric Function3 : Trigonometry  Operator=tan
  Trigonometric Function6 : Trigonometry
  Trigonometric Function8 : Trigonometry
  strap_down_matrix : Outport
  wires:
  Gain1/1 -> Mux1/3
  Matrix Concatenate/1 -> strap_down_matrix/1
  Mux/1 -> Reshape/1
  Product1/1 -> Mux/3
  Reshape1/1 -> Matrix Concatenate/2
  Constant6/1 -> Mux2/1
  Reshape/1 -> Matrix Concatenate/1
  Constant3/1 -> Mux1/1
  Trigonometric Function4/1 -> Mux1/2
  Trigonometric Function/1 -> Product/1
  Reshape2/1 -> Matrix Concatenate/3
  theta/1 -> Trigonometric Function3/1, Trigonometric Function11/1, Trigonometric Function9/1, Trigonometric Function1/1  "theta"
  Trigonometric Function3/1 -> Product1/2
  Trigonometric Function2/1 -> Product1/1
  Product/1 -> Mux/2
  Divide1/1 -> Mux2/3
  Trigonometric Function9/1 -> Divide2/2
  Trigonometric Function6/1 -> Gain1/1
  Mux2/1 -> Reshape2/1
  Trigonometric Function8/1 -> Divide2/1
  Trigonometric Function1/1 -> Product/2
  Mux1/1 -> Reshape1/1
  Trigonometric Function10/1 -> Divide1/1
  Trigonometric Function11/1 -> Divide1/2
  Divide2/1 -> Mux2/2
  Constant/1 -> Mux/1
  phi/1 -> Trigonometric Function10/1, Trigonometric Function8/1, Trigonometric Function6/1, Trigonometric Function4/1, Trigonometric Function2/1, Trigonometric Function/1  "phi"

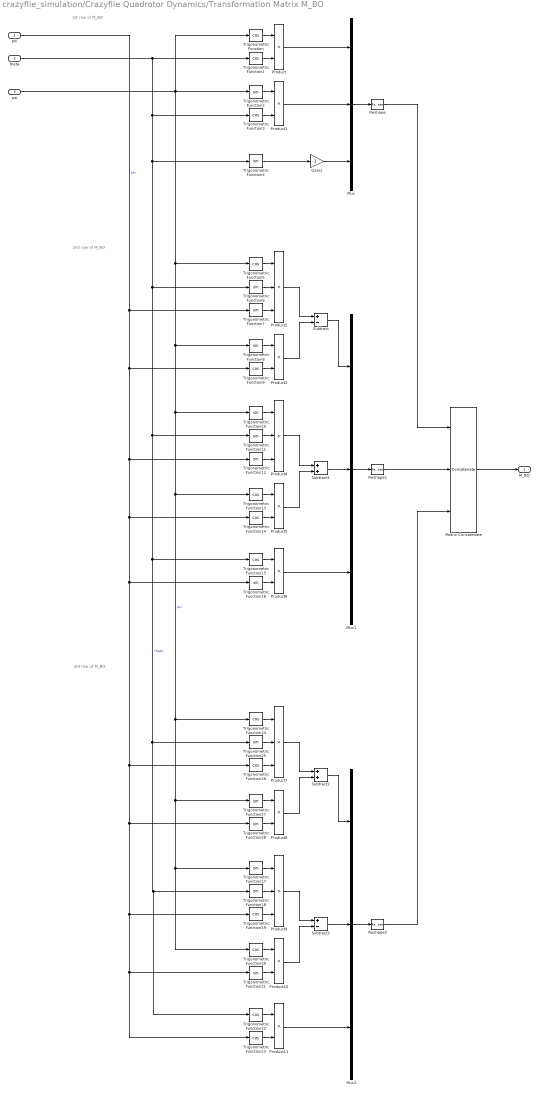
== system crazyflie_simulation/Crazyflie Quadrotor Dynamics/Transformation Matrix M_BO ==
  note: 3rd row of M_BO
  note: 2nd row of M_BO
  note: 1st row of M_BO
  phi : Inport
  theta : Inport  Port=2
  psi : Inport  Port=3
  Gain1 : Gain  Gain=-1
  Matrix Concatenate : Concatenate  NumInputs=3  Mode=Multidimensional array
  Mux : Mux  Inputs=3
  Mux1 : Mux  Inputs=3
  Mux2 : Mux  Inputs=3
  Product{,1,3,5..6,8,10..11} (8 alike) : Product
  Product{2,4,7,9} (4 alike) : Product  Inputs=3
  Reshape : Reshape  OutputDimensionality=Row vector (2-D)
  Reshape1 : Reshape  OutputDimensionality=Row vector (2-D)
  Reshape2 : Reshape  OutputDimensionality=Row vector (2-D)
  Subtract : Sum  Inputs=+-
  Subtract1 : Sum
  Subtract2 : Sum
  Subtract3 : Sum  Inputs=+-
  Trigonometric Function{,1,3,5,9,13..15,19..20,22..24,26} (14 alike) : Trigonometry  Operator=cos
  Trigonometric Function{2,4,6..8,10..12,16..18,21,25,27..28} (15 alike) : Trigonometry
  M_BO : Outport
  wires:
  Gain1/1 -> Mux/3
  Trigonometric Function/1 -> Product/1
  Trigonometric Function1/1 -> Product/2
  psi/1 -> Trigonometric Function20/1, Trigonometric Function17/1, Trigonometric Function27/1, Trigonometric Function24/1, Trigonometric Function13/1, Trigonometric Function10/1, Trigonometric Function8/1, Trigonometric Function5/1, Trigonometric Function/1, Trigonometric Function2/1  "psi"
  Trigonometric Function3/1 -> Product1/2
  Trigonometric Function2/1 -> Product1/1
  Product/1 -> Mux/1
  Product1/1 -> Mux/2
  Trigonometric Function4/1 -> Gain1/1
  Mux/1 -> Reshape/1
  Reshape/1 -> Matrix Concatenate/1
  Trigonometric Function5/1 -> Product2/1
  Trigonometric Function6/1 -> Product2/2
  theta/1 -> Trigonometric Function22/1, Trigonometric Function18/1, Trigonometric Function25/1, Trigonometric Function15/1, Trigonometric Function11/1, Trigonometric Function6/1, Trigonometric Function4/1, Trigonometric Function3/1, Trigonometric Function1/1  "theta"
  Trigonometric Function7/1 -> Product2/3
  phi/1 -> Trigonometric Function23/1, Trigonometric Function21/1, Trigonometric Function19/1, Trigonometric Function28/1, Trigonometric Function26/1, Trigonometric Function16/1, Trigonometric Function14/1, Trigonometric Function12/1, Trigonometric Function9/1, Trigonometric Function7/1  "phi"
  Trigonometric Function8/1 -> Product3/1
  Trigonometric Function9/1 -> Product3/2
  Product2/1 -> Subtract/1
  Product3/1 -> Subtract/2
  Product5/1 -> Subtract1/2
  Product4/1 -> Subtract1/1
  Trigonometric Function14/1 -> Product5/2
  Trigonometric Function13/1 -> Product5/1
  Trigonometric Function12/1 -> Product4/3
  Trigonometric Function11/1 -> Product4/2
  Trigonometric Function10/1 -> Product4/1
  Trigonometric Function16/1 -> Product6/2
  Trigonometric Function15/1 -> Product6/1
  Subtract/1 -> Mux1/1
  Product6/1 -> Mux1/3
  Subtract1/1 -> Mux1/2
  Mux1/1 -> Reshape1/1
  Reshape1/1 -> Matrix Concatenate/2
  Reshape2/1 -> Matrix Concatenate/3
  Mux2/1 -> Reshape2/1
  Subtract3/1 -> Mux2/2
  Product11/1 -> Mux2/3
  Subtract2/1 -> Mux2/1
  Trigonometric Function22/1 -> Product11/1
  Trigonometric Function23/1 -> Product11/2
  Trigonometric Function17/1 -> Product9/1
  Trigonometric Function18/1 -> Product9/2
  Trigonometric Function19/1 -> Product9/3
  Trigonometric Function20/1 -> Product10/1
  Trigonometric Function21/1 -> Product10/2
  Product9/1 -> Subtract3/1
  Product10/1 -> Subtract3/2
  Product8/1 -> Subtract2/2
  Product7/1 -> Subtract2/1
  Trigonometric Function28/1 -> Product8/2
  Trigonometric Function27/1 -> Product8/1
  Trigonometric Function26/1 -> Product7/3
  Trigonometric Function25/1 -> Product7/2
  Trigonometric Function24/1 -> Product7/1
  Matrix Concatenate/1 -> M_BO/1

== matlab function crazyflie_simulation/Pseudoinverse of u  ==
  data: u input; y output size=[3 3]
function y = fcn(u)

y = pinv(u);

== matlab function crazyflie_simulation/Pseudoinverse of u ==
  data: u input; y output
function y = fcn(u)

y = pinv(u);
